simulink model "PID"  (R2020b)
settings: Solver=ode45  StartTime=0.0  StopTime=3  RelTol=1e-4
undefined symbols (not defined in the file or in its folder): daq, drv, gbox, mld, mot, pid, rads2rpm, sens
settings Model: Creator=Utente  LastModifiedBy=Utente
settings SolverCC: ZeroCrossAlgorithm=Adaptive
settings DataIOCC: ReturnWorkspaceOutputs=off
settings DebuggingCC: IgnoredZcDiagnostic=none

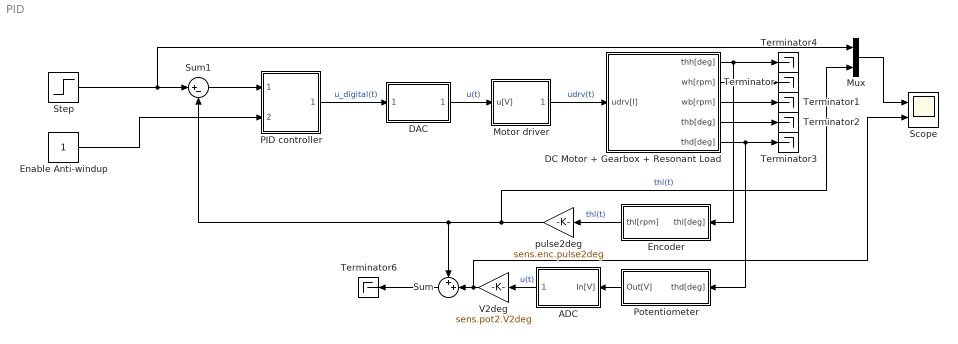
== system PID ==
  ADC : Subsystem
  DAC : Subsystem
  DC Motor + Gearbox + Resonant Load : Subsystem
  Enable Anti-windup : Constant
  Encoder : Subsystem
  Motor driver : Subsystem
  Mux : Mux  Inputs=2
  "PID controller " : Subsystem
  Potentiometer : Subsystem
  Scope : Scope  NumInputPorts=2
  Step : Step  Time=0  After=50  SampleTime=0
  Sum : Sum  Inputs=++|
  Sum1 : Sum  Inputs=|+-
  Terminator{,1..4,6} (6 alike) : Terminator
  V2deg : Gain  Gain=sens.pot2.V2deg
  pulse2deg : Gain  Gain=sens.enc.pulse2deg
  wires:
  DC Motor + Gearbox + Resonant Load/5(thd[deg]) -> Terminator3/1, Potentiometer/1(thd[deg])
  DC Motor + Gearbox + Resonant Load/1(thh[deg]) -> Terminator4/1, Encoder/1(thl[deg])
  DC Motor + Gearbox + Resonant Load/2(wh[rpm]) -> Terminator/1
  DC Motor + Gearbox + Resonant Load/3(wb[rpm]) -> Terminator1/1
  DC Motor + Gearbox + Resonant Load/4(thb[deg]) -> Terminator2/1
  Encoder/1(thl[rpm]) -> pulse2deg/1  "thl(t)"
  V2deg/1 -> Scope/2, Sum/2
  pulse2deg/1 -> Mux/2, Sum1/2, Sum/1  "thl(t)"
  Sum/1 -> Terminator6/1
  Motor driver/1(udrv[I]) -> DC Motor + Gearbox + Resonant Load/1(udrv[I])  "udrv(t)"
  DAC/1(Out[V]) -> Motor driver/1(u[V])  "u(t)"
  ADC/1(Out[V]) -> V2deg/1  "u(t)"
  Potentiometer/1(Out[V]) -> ADC/1(In[V])
  "PID controller "/1(u[rad]) -> DAC/1(In[rad])  "u_digital(t)"
  Sum1/1 -> "PID controller "/1(e[deg])
  Step/1 -> Mux/1, Sum1/1
  Enable Anti-windup/1 -> "PID controller "/2(aw_enable)
  Mux/1 -> Scope/1

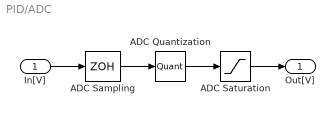
== system PID/ADC ==
  In[V] : Inport
  ADC Quantization : Quantizer  QuantizationInterval=daq.adc.q
  ADC Sampling : ZeroOrderHold  SampleTime=daq.adc.T_s
  ADC Saturation : Saturate  UpperLimit=daq.adc.vdd  LowerLimit=daq.adc.vss
  Out[V] : Outport
  wires:
  ADC Quantization/1 -> ADC Saturation/1
  ADC Sampling/1 -> ADC Quantization/1
  ADC Saturation/1 -> Out[V]/1
  In[V]/1 -> ADC Sampling/1

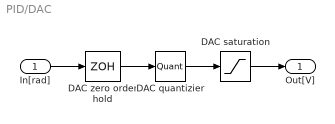
== system PID/DAC ==
  In[rad] : Inport
  DAC quantizier : Quantizer  QuantizationInterval=daq.dac.q
  DAC saturation : Saturate  UpperLimit=daq.dac.vdd  LowerLimit=daq.dac.vss
  DAC zero order hold : ZeroOrderHold  SampleTime=daq.dac.T_s
  Out[V] : Outport
  wires:
  DAC quantizier/1 -> DAC saturation/1
  DAC zero order hold/1 -> DAC quantizier/1
  DAC saturation/1 -> Out[V]/1
  In[rad]/1 -> DAC zero order hold/1

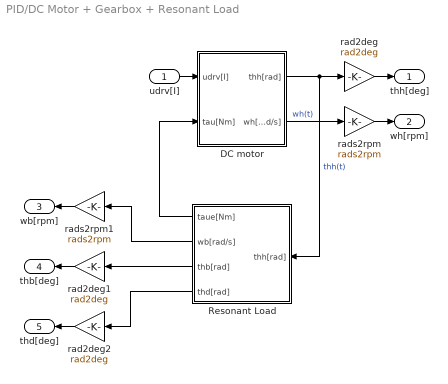
== system PID/DC Motor + Gearbox + Resonant Load ==
  udrv[I] : Inport
  DC motor : Subsystem
  Resonant Load : Subsystem
  rad2deg : Gain  Gain=rad2deg
  rad2deg1 : Gain  Gain=rad2deg
  rad2deg2 : Gain  Gain=rad2deg
  rads2rpm : Gain  Gain=rads2rpm
  rads2rpm1 : Gain  Gain=rads2rpm
  thh[deg] : Outport
  wh[rpm] : Outport  Port=2
  wb[rpm] : Outport  Port=3
  thb[deg] : Outport  Port=4
  thd[deg] : Outport  Port=5
  wires:
  rad2deg2/1 -> thd[deg]/1
  rad2deg1/1 -> thb[deg]/1
  DC motor/1(thh[rad]) -> Resonant Load/1(thh[rad]), rad2deg/1  "thh(t)"
  Resonant Load/2(wb[rad/s]) -> rads2rpm1/1
  Resonant Load/4(thd[rad]) -> rad2deg2/1
  Resonant Load/3(thb[rad]) -> rad2deg1/1
  DC motor/2(wh[rad/s]) -> rads2rpm/1  "wh(t)"
  udrv[I]/1 -> DC motor/1(udrv[I])
  rad2deg/1 -> thh[deg]/1
  rads2rpm/1 -> wh[rpm]/1
  rads2rpm1/1 -> wb[rpm]/1
  Resonant Load/1(taue[Nm]) -> DC motor/2(tau[Nm])

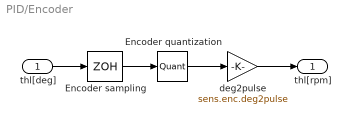
== system PID/Encoder ==
  thl[deg] : Inport
  Encoder quantization : Quantizer  QuantizationInterval=sens.enc.q
  Encoder sampling : ZeroOrderHold  SampleTime=sens.enc.T_s
  deg2pulse : Gain  Gain=sens.enc.deg2pulse
  thl[rpm] : Outport
  wires:
  Encoder quantization/1 -> deg2pulse/1
  deg2pulse/1 -> thl[rpm]/1
  Encoder sampling/1 -> Encoder quantization/1
  thl[deg]/1 -> Encoder sampling/1

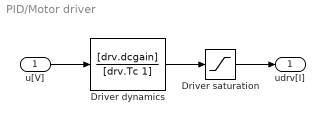
== system PID/Motor driver ==
  u[V] : Inport
  Driver dynamics : TransferFcn  Numerator=[drv.dcgain]  Denominator=[drv.Tc 1]
  Driver saturation : Saturate  UpperLimit=drv.vp  LowerLimit=drv.vm
  udrv[I] : Outport
  wires:
  Driver saturation/1 -> udrv[I]/1
  Driver dynamics/1 -> Driver saturation/1
  u[V]/1 -> Driver dynamics/1

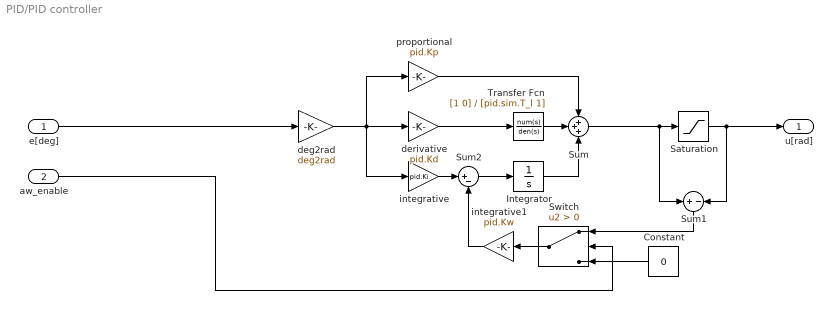
== system PID/PID controller  ==
  e[deg] : Inport  Unit=deg
  aw_enable : Inport  Port=2  Unit=deg
  Constant : Constant  Value=0
  Integrator : Integrator
  Saturation : Saturate  UpperLimit=daq.dac.vdd  LowerLimit=daq.dac.vss
  Sum : Sum  Inputs=+++
  Sum1 : Sum  Inputs=+|-
  Sum2 : Sum  Inputs=|+-
  Switch : Switch  Criteria=u2 > Threshold
  Transfer Fcn : TransferFcn  Numerator=[1 0]  Denominator=[pid.sim.T_l 1]
  deg2rad : Gain  Gain=deg2rad
  derivative : Gain  Gain=pid.Kd
  integrative : Gain  Gain=pid.Ki
  integrative1 : Gain  Gain=pid.Kw
  proportional : Gain  Gain=pid.Kp
  u[rad] : Outport
  wires:
  deg2rad/1 -> integrative/1, derivative/1, proportional/1
  proportional/1 -> Sum/1
  Saturation/1 -> u[rad]/1, Sum1/2
  integrative/1 -> Sum2/1
  Sum2/1 -> Integrator/1
  integrative1/1 -> Sum2/2
  Integrator/1 -> Sum/3
  Transfer Fcn/1 -> Sum/2
  derivative/1 -> Transfer Fcn/1
  aw_enable/1 -> Switch/2
  Constant/1 -> Switch/3
  Switch/1 -> integrative1/1
  Sum1/1 -> Switch/1
  Sum/1 -> Saturation/1, Sum1/1
  e[deg]/1 -> deg2rad/1

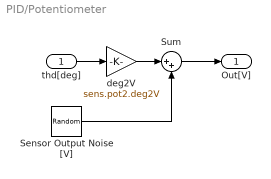
== system PID/Potentiometer ==
  thd[deg] : Inport
  Sensor Output Noise [V] : RandomNumber  Variance=sens.pot2.noise.var  SampleTime=0.1
  Sum : Sum  Inputs=|++
  deg2V : Gain  Gain=sens.pot2.deg2V
  Out[V] : Outport
  wires:
  thd[deg]/1 -> deg2V/1
  Sensor Output Noise [V]/1 -> Sum/2
  deg2V/1 -> Sum/1
  Sum/1 -> Out[V]/1

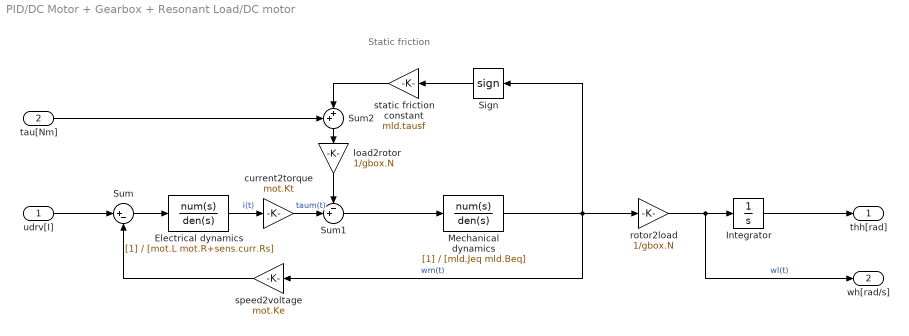
== system PID/DC Motor + Gearbox + Resonant Load/DC motor ==
  note: Static friction
  udrv[I] : Inport  Unit=V
  tau[Nm] : Inport  Port=2  Unit=V
  Electrical dynamics : TransferFcn  Denominator=[mot.L mot.R+sens.curr.Rs]
  Integrator : Integrator
  Mechanical dynamics : TransferFcn  Denominator=[mld.Jeq mld.Beq]
  Sign : Signum  ZeroCross=off
  Sum : Sum  Inputs=|+-
  Sum1 : Sum  Inputs=-+|
  Sum2 : Sum  Inputs=++|
  current2torque : Gain  Gain=mot.Kt
  load2rotor : Gain  Gain=1/gbox.N
  rotor2load : Gain  Gain=1/gbox.N
  speed2voltage : Gain  Gain=mot.Ke
  static friction constant : Gain  Gain=mld.tausf
  thh[rad] : Outport  Unit=deg
  wh[rad/s] : Outport  Port=2  Unit=rpm
  wires:
  load2rotor/1 -> Sum1/1
  Mechanical dynamics/1 -> Sign/1, rotor2load/1, speed2voltage/1  "wm(t)"
  Sign/1 -> static friction constant/1
  current2torque/1 -> Sum1/2  "taum(t)"
  Sum1/1 -> Mechanical dynamics/1
  speed2voltage/1 -> Sum/2
  rotor2load/1 -> wh[rad/s]/1, Integrator/1  "wl(t)"
  Electrical dynamics/1 -> current2torque/1  "i(t)"
  Sum/1 -> Electrical dynamics/1
  Integrator/1 -> thh[rad]/1
  udrv[I]/1 -> Sum/1
  static friction constant/1 -> Sum2/2
  Sum2/1 -> load2rotor/1
  tau[Nm]/1 -> Sum2/1

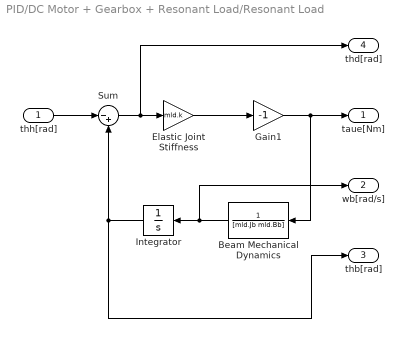
== system PID/DC Motor + Gearbox + Resonant Load/Resonant Load ==
  thh[rad] : Inport
  Beam Mechanical Dynamics : TransferFcn  Denominator=[mld.Jb mld.Bb]
  Elastic Joint Stiffness : Gain  Gain=mld.k
  Gain1 : Gain  Gain=-1
  Integrator : Integrator
  Sum : Sum  Inputs=|-+
  taue[Nm] : Outport
  wb[rad/s] : Outport  Port=2
  thb[rad] : Outport  Port=3
  thd[rad] : Outport  Port=4
  wires:
  Beam Mechanical Dynamics/1 -> wb[rad/s]/1, Integrator/1
  Elastic Joint Stiffness/1 -> Gain1/1
  Gain1/1 -> taue[Nm]/1, Beam Mechanical Dynamics/1
  thh[rad]/1 -> Sum/1
  Integrator/1 -> thb[rad]/1, Sum/2
  Sum/1 -> thd[rad]/1, Elastic Joint Stiffness/1
